simulink model "ESKF"  (R2022b)
settings: Solver=VariableStepAuto  StartTime=0.0  StopTime=10.0  RelTol=1e-3
settings Model: Creator=89565  LastModifiedBy=89565

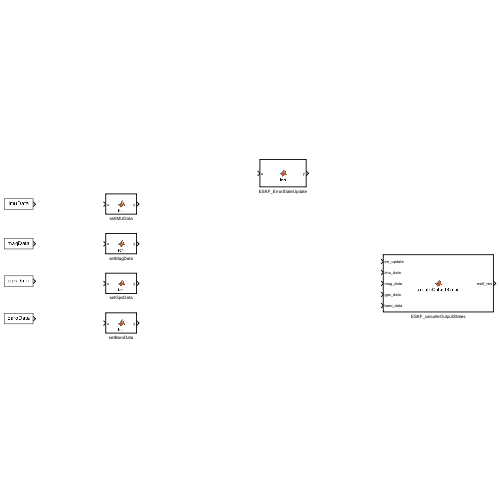
[thumbnail: Simulink's stored preview of the top-level diagram]
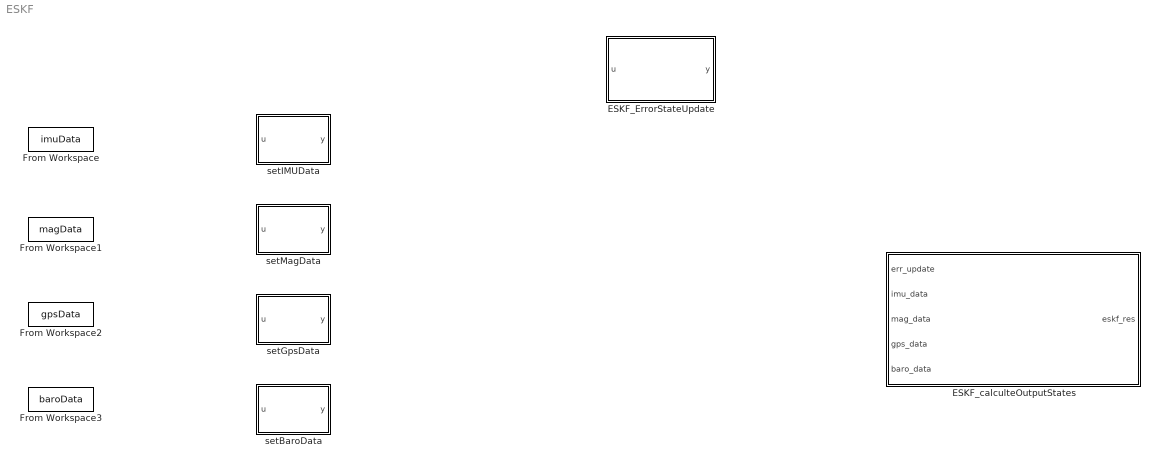
== system ESKF ==
  ESKF_ErrorStateUpdate : MATLAB Function  TreatAsAtomicUnit=on
  ESKF_calculteOutputStates : MATLAB Function  TreatAsAtomicUnit=on
  From Workspace : FromWorkspace  VariableName=imuData
  From Workspace1 : FromWorkspace  VariableName=magData
  From Workspace2 : FromWorkspace  VariableName=gpsData
  From Workspace3 : FromWorkspace  VariableName=baroData
  setBaroData : MATLAB Function  TreatAsAtomicUnit=on
  setGpsData : MATLAB Function  TreatAsAtomicUnit=on
  setIMUData : MATLAB Function  TreatAsAtomicUnit=on
  setMagData : MATLAB Function  TreatAsAtomicUnit=on

== matlab function ESKF/setIMUData ==
  data: u input; y output
function y = fcn(u)

y = u;

== matlab function ESKF/ESKF_calculteOutputStates ==
  data: err_update input; eskf_res output; imu_data input; mag_data input; gps_data input; baro_data input
function eskf_res = calculteOutputStates(err_update,imu_data,mag_data,gps_data,baro_data)




eskf_res = u;

== matlab function ESKF/setMagData ==
  data: u input; y output
function y = fcn(u)

y = u;

== matlab function ESKF/setGpsData ==
  data: u input; y output
function y = fcn(u)

y = u;

== matlab function ESKF/setBaroData ==
  data: u input; y output
function y = fcn(u)

y = u;

== matlab function ESKF/ESKF_ErrorStateUpdate ==
  data: u input; y output
function y = fcn(u)

y = u;
